simulink model "MFWF_plant"  (R2021a)
settings: Solver=FixedStepAuto  StartTime=0  StopTime=10.0  MaxStep=0.1  RelTol=1e-3  EnableMultiTasking=on
InitFcn:
  | aero_control_dynamics_config
model workspace (MAT data in the model file):
  CG = [0 0 0]
  g = [0 0 -9.81]
  t_sensor = 0.02
undefined symbols (not defined in the file or in its folder): DiscIntNeverNeededParam
libraries: shared6dof x1, aerolibnav x1, aerolibcommonsys x1
settings Model: ModifiedByFormat=The MathWorks Inc.  OrderedModelArguments=off  Creator=The MathWorks, Inc.  LastModifiedBy=The MathWorks Inc.
settings SolverCC: AlgebraicLoopSolver=TrustRegion
settings DataIOCC: SaveFormat=StructureWithTime  ReturnWorkspaceOutputs=off
settings OptimizationCC: BlockReduction=off  DefaultParameterBehavior=Inlined  BufferReuse=off  ExpressionDepthLimit=2147483647  LifeSpan=1
settings DebuggingCC: AlgebraicLoopMsg=none  UnderspecifiedInitializationDetection=Classic  MergeDetectMultiDrivingBlocksExec=none  FcnCallInpInsideContextMsg=warning  UnconnectedInputMsg=none  UnconnectedOutputMsg=none  UnconnectedLineMsg=none  AllowSymbolicDim=off  StateNameClashWarn=warning  SFUnexpectedBacktrackingDiag=warning  SFNoUnconditionalDefaultTransitionDiag=warning  SFExecutionAtInitializationDiag=none  SFMachineParentedDataDiag=warning  ArithmeticOperatorsInVariantConditions=warning
settings HardwareCC: ProdBitPerPointer=32  ProdBitPerSizeT=32  ProdBitPerPtrDiffT=32  ProdLargestAtomicFloat=None  ProdIntDivRoundTo=Undefined  ProdEndianess=Unspecified  ProdWordSize=32  ProdHWDeviceType=32-bit Generic
settings ModelReferenceCC: PropagateSignalLabelsOutOfModel=off
settings SFSimCC: SimUseLocalCustomCode=off  CustomCodeUndefinedFunction=UseInterfaceOnly
settings RTWCC: RTWUseLocalCustomCode=off
settings CodeAppCC: StateflowObjectComments=on
settings GRTTargetCC: TargetLangStandard=C89/C90 (ANSI)  CombineOutputUpdateFcns=off  GRTInterface=on
settings ConfigComp: CovMetricSettings=dw  CovSaveCumulativeToWorkspaceVar=on  CovSaveSingleToWorkspaceVar=on  CovExternalEMLEnable=off  CovSFcnEnable=off

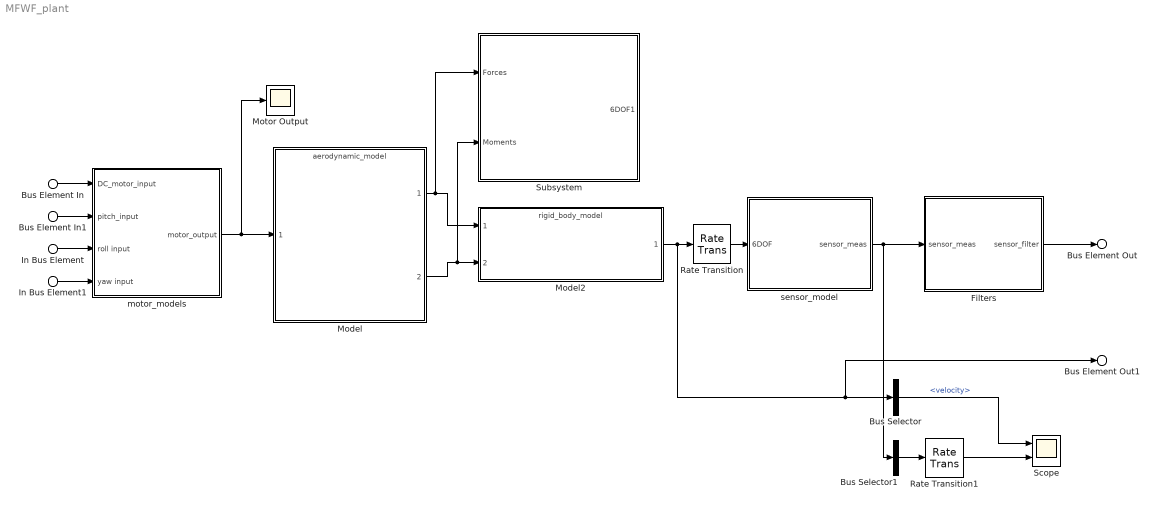
== system MFWF_plant ==
  Bus Element In : Inport  PortName=motor_input  Element=flapping_freq
  Bus Element In1 : Inport  PortName=motor_input  Element=pitch
  In Bus Element : Inport  PortName=motor_input  Element=yaw
  In Bus Element1 : Inport  PortName=motor_input  Element=roll
  Bus Selector : BusSelector  OutputSignals=inertial.velocity
  Bus Selector1 : BusSelector  OutputSignals=Vx,Vy,Vz  OutputAsBus=on
  Filters : Subsystem
  Model : ModelReference  ModelNameDialog=aerodynamic_model  SimulationMode=Normal  ModelReferenceVersion=8.16
  Model2 : ModelReference  ModelNameDialog=rigid_body_model  SimulationMode=Normal  ModelReferenceVersion=8.27
  Motor Output : Scope
  Rate Transition : RateTransition
  Rate Transition1 : RateTransition
  Scope : Scope  NumInputPorts=2
  Subsystem : Subsystem
  motor_models : Subsystem
  sensor_model : Subsystem
  Bus Element Out : Outport  PortName=sensor
  Bus Element Out1 : Outport  Port=2  PortName=6DOF
  wires:
  Model/1 -> Subsystem/1(Forces), Model2/1
  Model/2 -> Subsystem/2(Moments), Model2/2
  In Bus Element/1 -> motor_models/3(roll input)
  In Bus Element1/1 -> motor_models/4(yaw input)
  Bus Element In/1 -> motor_models/1(DC_motor_input)
  Bus Element In1/1 -> motor_models/2(pitch_input)
  motor_models/1(motor_output) -> Motor Output/1, Model/1
  sensor_model/1(sensor_meas) -> Bus Selector1/1, Filters/1(sensor_meas)
  Rate Transition/1 -> sensor_model/1(6DOF)
  Filters/1(sensor_filter) -> Bus Element Out/1
  Model2/1 -> Bus Selector/1, Bus Element Out1/1, Rate Transition/1
  Bus Selector/1 -> Scope/1  "<velocity>"
  Bus Selector1/1 -> Rate Transition1/1
  Rate Transition1/1 -> Scope/2

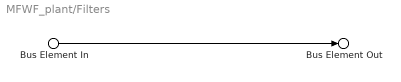
== system MFWF_plant/Filters ==
  Bus Element In : Inport  PortName=sensor_meas
  Bus Element Out : Outport  PortName=sensor_filter
  wires:
  Bus Element In/1 -> Bus Element Out/1

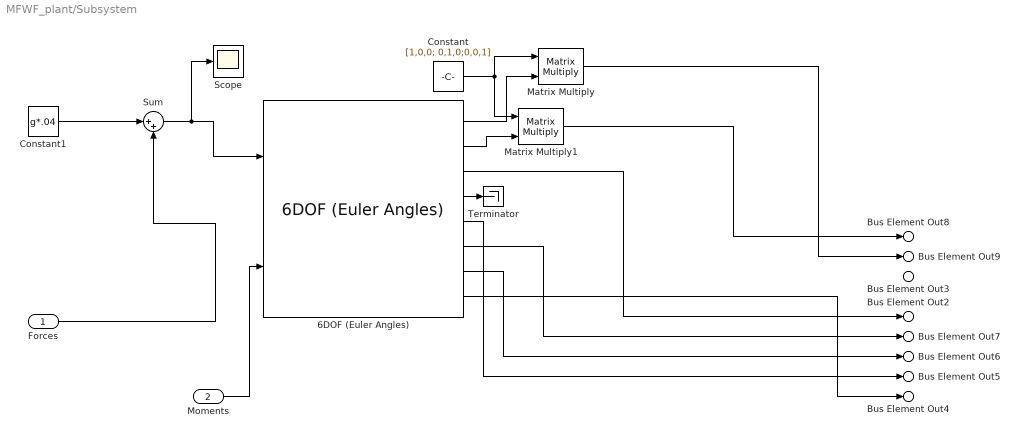
== system MFWF_plant/Subsystem ==
  Forces : Inport
  Moments : Inport  Port=2
  6DOF (Euler Angles) : shared6dof/6DOF (Euler Angles)  units=Metric (MKS)  mtype=Fixed  rep=Euler Angles  xme_0=[0 0 0]  Vm_0=[0 0 0]  eul_0=[0 0 0]  pm_0=[0 0 0]  mass_0=0.04  mass_e=0.5  mass_f=2.0  inertia=[0.0034 0.0000 0.0000; 0.0000 0.0010 0.0000; 0.0000 0.0000 0.0026]  inertia_e=eye(3)  inertia_f=2*eye(3)  k_quat=1.0  vre_flag=on  abi_flag=off  aMode=0  xme_statename=''  Vm_statename=''  eul_statename=''  quat_statename=''  pm_statename=''  mass_statename=''
      settings: SourceProductBaseCode=AE,PW,DR,MT,UV,VE
  Constant : Constant  Value=[1,0,0; 0,1,0;0,0,1]
  Constant1 : Constant  Value=g*.04
  Matrix Multiply : Product  Multiplication=Matrix(*)
  Matrix Multiply1 : Product  Multiplication=Matrix(*)
  Scope : Scope
  Sum : Sum  Inputs=|++
  Terminator : Terminator
  Bus Element Out2 : Outport  PortName=6DOF1  Element=body.angles
  Bus Element Out5 : Outport  PortName=6DOF1  Element=body.velocity
  Bus Element Out4 : Outport  PortName=6DOF1  Element=body.acceleration
  Bus Element Out6 : Outport  PortName=6DOF1  Element=body.angularAccel
  Bus Element Out7 : Outport  PortName=6DOF1  Element=body.angularRate
  Bus Element Out3 : Outport  PortName=6DOF1  Element=inertial.angularRate
  Bus Element Out8 : Outport  PortName=6DOF1  Element=inertial.position
  Bus Element Out9 : Outport  PortName=6DOF1  Element=inertial.velocity
  wires:
  Forces/1 -> Sum/2
  Moments/1 -> 6DOF (Euler Angles)/2
  6DOF (Euler Angles)/8 -> Bus Element Out4/1
  Matrix Multiply1/1 -> Bus Element Out8/1
  Matrix Multiply/1 -> Bus Element Out9/1
  6DOF (Euler Angles)/3 -> Bus Element Out2/1
  6DOF (Euler Angles)/6 -> Bus Element Out7/1
  6DOF (Euler Angles)/7 -> Bus Element Out6/1
  6DOF (Euler Angles)/5 -> Bus Element Out5/1
  6DOF (Euler Angles)/2 -> Matrix Multiply1/2
  Constant/1 -> Matrix Multiply/1, Matrix Multiply1/1
  6DOF (Euler Angles)/1 -> Matrix Multiply/2
  6DOF (Euler Angles)/4 -> Terminator/1
  Constant1/1 -> Sum/1
  Sum/1 -> Scope/1, 6DOF (Euler Angles)/1

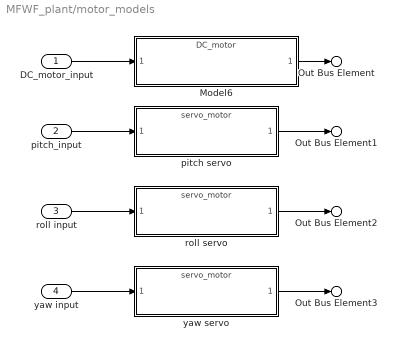
== system MFWF_plant/motor_models ==
  DC_motor_input : Inport
  pitch_input : Inport  Port=2
  roll input : Inport  Port=3
  yaw input : Inport  Port=4
  Model6 : ModelReference  ModelNameDialog=DC_motor  SimulationMode=Normal  ModelReferenceVersion=8.10
  pitch servo : ModelReference  ModelNameDialog=servo_motor  SimulationMode=Normal  ModelReferenceVersion=8.10
  roll servo : ModelReference  ModelNameDialog=servo_motor  SimulationMode=Normal  ModelReferenceVersion=8.10
  yaw servo : ModelReference  ModelNameDialog=servo_motor  SimulationMode=Normal  ModelReferenceVersion=8.10
  Out Bus Element : Outport  PortName=motor_output  Element=flapping_freq
  Out Bus Element1 : Outport  PortName=motor_output  Element=pitch
  Out Bus Element3 : Outport  PortName=motor_output  Element=roll
  Out Bus Element2 : Outport  PortName=motor_output  Element=yaw
  wires:
  roll servo/1 -> Out Bus Element2/1
  pitch servo/1 -> Out Bus Element1/1
  yaw servo/1 -> Out Bus Element3/1
  pitch_input/1 -> pitch servo/1
  roll input/1 -> roll servo/1
  yaw input/1 -> yaw servo/1
  DC_motor_input/1 -> Model6/1
  Model6/1 -> Out Bus Element/1

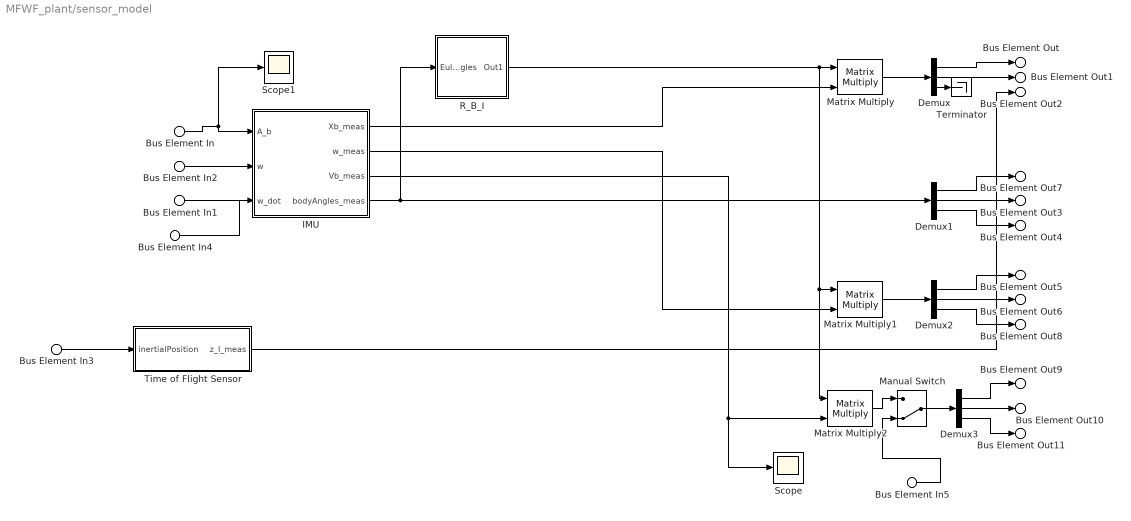
== system MFWF_plant/sensor_model ==
  Bus Element In : Inport  PortName=6DOF  Element=body.acceleration
  Bus Element In1 : Inport  PortName=6DOF  Element=body.angularAccel
  Bus Element In2 : Inport  PortName=6DOF  Element=body.angularRate
  Bus Element In4 : Inport  PortName=6DOF  Element=body.angles
  Bus Element In3 : Inport  PortName=6DOF  Element=inertial.position
  Bus Element In5 : Inport  PortName=6DOF  Element=inertial.velocity
  Demux{,1..3} (4 alike) : Demux  Outputs=3
  IMU : Subsystem
  Manual Switch : ManualSwitch  CurrentSetting=0
  Matrix Multiply : Product  Multiplication=Matrix(*)
  Matrix Multiply1 : Product  Multiplication=Matrix(*)
  Matrix Multiply2 : Product  Multiplication=Matrix(*)
  R_B_I : Subsystem
  Scope : Scope
  Scope1 : Scope
  Terminator : Terminator
  Time of Flight Sensor : Subsystem
  Bus Element Out : Outport  PortName=sensor_meas  Element=x
  Bus Element Out1 : Outport  PortName=sensor_meas  Element=y
  Bus Element Out7 : Outport  PortName=sensor_meas  Element=phi
  Bus Element Out3 : Outport  PortName=sensor_meas  Element=theta
  Bus Element Out4 : Outport  PortName=sensor_meas  Element=psi
  Bus Element Out5 : Outport  PortName=sensor_meas  Element=p
  Bus Element Out6 : Outport  PortName=sensor_meas  Element=q
  Bus Element Out8 : Outport  PortName=sensor_meas  Element=r
  Bus Element Out9 : Outport  PortName=sensor_meas  Element=Vx
  Bus Element Out10 : Outport  PortName=sensor_meas  Element=Vy
  Bus Element Out11 : Outport  PortName=sensor_meas  Element=Vz
  Bus Element Out2 : Outport  PortName=sensor_meas  Element=z
  wires:
  R_B_I/1(Out1) -> Matrix Multiply1/1, Matrix Multiply2/1, Matrix Multiply/1
  IMU/3(Vb_meas) -> Scope/1, Matrix Multiply2/2
  IMU/2(w_meas) -> Matrix Multiply1/2
  Matrix Multiply1/1 -> Demux2/1
  IMU/1(Xb_meas) -> Matrix Multiply/2
  Matrix Multiply/1 -> Demux/1
  IMU/4(bodyAngles_meas) -> Demux1/1, R_B_I/1(Euler_angles)
  Bus Element In1/1 -> IMU/3(w_dot)
  Time of Flight Sensor/1(z_I_meas) -> Bus Element Out2/1
  Bus Element In3/1 -> Time of Flight Sensor/1(inertialPosition)
  Demux1/2 -> Bus Element Out3/1
  Demux1/3 -> Bus Element Out4/1
  Demux2/2 -> Bus Element Out6/1
  Demux/2 -> Bus Element Out1/1
  Demux1/1 -> Bus Element Out7/1
  Demux2/1 -> Bus Element Out5/1
  Demux/1 -> Bus Element Out/1
  Demux3/2 -> Bus Element Out10/1
  Demux3/1 -> Bus Element Out9/1
  Demux2/3 -> Bus Element Out8/1
  Bus Element In/1 -> Scope1/1, IMU/1(A_b)
  Bus Element In2/1 -> IMU/2(w)
  Bus Element In4/1 -> ?
  Demux/3 -> Terminator/1
  Demux3/3 -> Bus Element Out11/1
  Manual Switch/1 -> Demux3/1
  Matrix Multiply2/1 -> Manual Switch/1
  Bus Element In5/1 -> Manual Switch/2

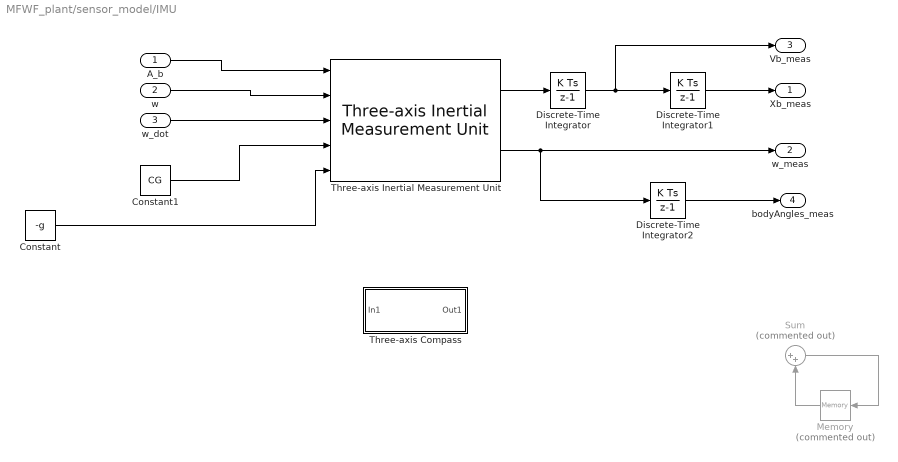
== system MFWF_plant/sensor_model/IMU ==
  A_b : Inport
  w : Inport  Port=2
  w_dot : Inport  Port=3
  Constant : Constant  Value=-g
  Constant1 : Constant  Value=CG
  Discrete-Time Integrator : DiscreteIntegrator  SampleTime=-1  ICPrevOutput=DiscIntNeverNeededParam  ICPrevScaledInput=DiscIntNeverNeededParam
  Discrete-Time Integrator1 : DiscreteIntegrator  SampleTime=-1  ICPrevOutput=DiscIntNeverNeededParam  ICPrevScaledInput=DiscIntNeverNeededParam
  Discrete-Time Integrator2 : DiscreteIntegrator  SampleTime=-1  ICPrevOutput=DiscIntNeverNeededParam  ICPrevScaledInput=DiscIntNeverNeededParam
  Memory : Memory  Commented=on  InheritSampleTime=on
  Sum : Sum  Commented=on  Inputs=|++
  Three-axis Compass : Subsystem
  Three-axis Inertial Measurement Unit : aerolibnav/Three-axis Inertial Measurement Unit  units=Metric (MKS)  imu=[0 0 0]  i_Ts=t_sensor  dtype_a=on  w_a=190  z_a=0.707  a_sf_cc=[1 0 0; 0 1 0; 0 0 1]  a_bias=[0 0 0]  a_sat="[-inf  -inf  -inf  inf inf inf]"  dtype_g=on  w_g=190  z_g=0.707  g_sf_cc=[1 0 0; 0 1 0; 0 0 1]  g_bias=[0 0 0]  g_sens=[0 0 0]  g_sat="[-inf  -inf  -inf  inf inf inf]"  i_rand=on  i_seeds=[23093 23094 23095 23096 23097 23098]  i_pow=[0.001 0.001 0.001 0.0001 0.0001 0.0001]
  Xb_meas : Outport
  w_meas : Outport  Port=2
  Vb_meas : Outport  Port=3
  bodyAngles_meas : Outport  Port=4
  wires:
  Constant1/1 -> Three-axis Inertial Measurement Unit/4
  Three-axis Inertial Measurement Unit/2 -> Discrete-Time Integrator2/1, w_meas/1
  w/1 -> Three-axis Inertial Measurement Unit/2
  w_dot/1 -> Three-axis Inertial Measurement Unit/3
  Three-axis Inertial Measurement Unit/1 -> Discrete-Time Integrator/1
  A_b/1 -> Three-axis Inertial Measurement Unit/1
  Discrete-Time Integrator/1 -> Discrete-Time Integrator1/1, Vb_meas/1
  Discrete-Time Integrator1/1 -> Xb_meas/1
  Sum/1 -> Memory/1
  Memory/1 -> Sum/2
  Discrete-Time Integrator2/1 -> bodyAngles_meas/1
  Constant/1 -> Three-axis Inertial Measurement Unit/5

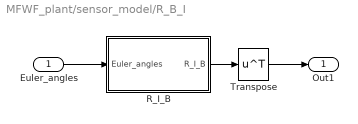
== system MFWF_plant/sensor_model/R_B_I ==
  Euler_angles : Inport
  R_I_B : Subsystem
  Transpose : Math  Operator=transpose  SaturateOnIntegerOverflow=on
  Out1 : Outport
  wires:
  Euler_angles/1 -> R_I_B/1(Euler_angles)
  Transpose/1 -> Out1/1
  R_I_B/1(R_I_B) -> Transpose/1

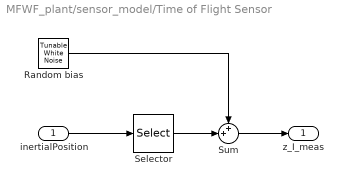
== system MFWF_plant/sensor_model/Time of Flight Sensor ==
  inertialPosition : Inport
  Random bias : aerolibcommonsys/Tunable White Noise  pwr=0.001  Ts=t_sensor  seed=1337
      settings: SourceProductBaseCode=AE
  Selector : Selector  InputPortWidth=3  IndexOptions=Index vector (dialog)  Indices=[3]  OutputSizes=1
  Sum : Sum  Inputs=++|
  z_I_meas : Outport
  wires:
  inertialPosition/1 -> Selector/1
  Random bias/1 -> Sum/1
  Sum/1 -> z_I_meas/1
  Selector/1 -> Sum/2

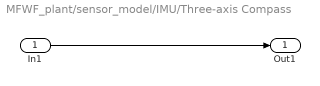
== system MFWF_plant/sensor_model/IMU/Three-axis Compass ==
  In1 : Inport
  Out1 : Outport
  wires:
  In1/1 -> Out1/1

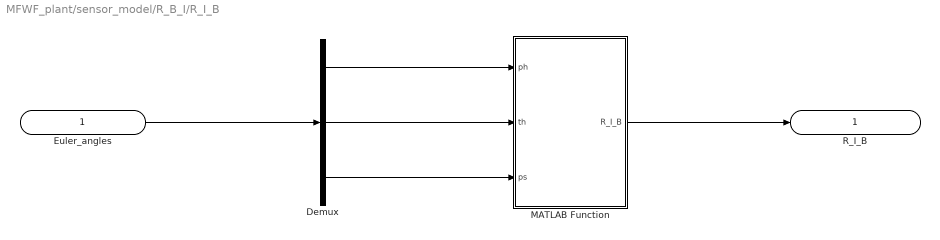
== system MFWF_plant/sensor_model/R_B_I/R_I_B ==
  Euler_angles : Inport
  Demux : Demux  Outputs=[1;1;1]
  MATLAB Function : MATLAB Function  TreatAsAtomicUnit=on
  R_I_B : Outport
  wires:
  MATLAB Function/1(R_I_B) -> R_I_B/1
  Demux/1 -> MATLAB Function/1(ph)
  Demux/3 -> MATLAB Function/3(ps)
  Demux/2 -> MATLAB Function/2(th)
  Euler_angles/1 -> Demux/1

== matlab function MFWF_plant/sensor_model/R_B_I/R_I_B/MATLAB Function ==
  data: ph input; R_I_B output; th input; ps input
function R_I_B = calc_R_I_B(ph, th, ps)

R_I_B = [cos(th)*cos(ps)              cos(th)*sin(ps)              -sin(th);
               sin(ph)*sin(th)*cos(ps)-cos(ph)*sin(ps)  sin(ph)*sin(th)*sin(ps)+cos(ph)*cos(ps)  sin(ph)*cos(th);
               cos(ph)*sin(th)*cos(ps)+sin(ph)*sin(ps)  cos(ph)*sin(th)*sin(ps)-sin(ph)*cos(ps)  cos(ph)*cos(th)];
end
